simulink model "SistemaMasaResorteAmortiguadorDobleMasa"  (R2019a)
settings: Solver=VariableStepAuto  StartTime=0.0  StopTime=50  RelTol=1e-3
settings Model: Creator=User  LastModifiedBy=User

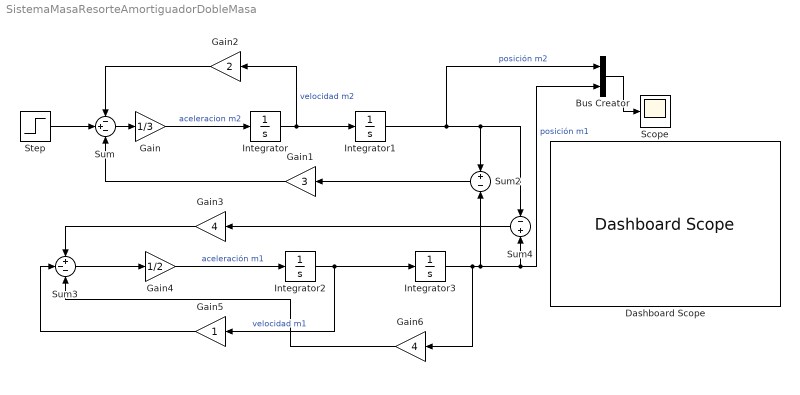
== system SistemaMasaResorteAmortiguadorDobleMasa ==
  Bus Creator : BusCreator  Inputs=2
  Dashboard Scope : DashboardScope
  Gain : Gain  Gain=1/3
  Gain1 : Gain  Gain=3
  Gain2 : Gain  Gain=2
  Gain3 : Gain  Gain=4
  Gain4 : Gain  Gain=1/2
  Gain5 : Gain
  Gain6 : Gain  Gain=4
  Integrator{,1..3} (4 alike) : Integrator
  Scope : Scope
  Step : Step  SampleTime=0
  Sum : Sum  Inputs=-+-
  Sum2 : Sum  Inputs=+-
  Sum3 : Sum  Inputs=+--
  Sum4 : Sum  Inputs=-+
  wires:
  Step/1 -> Sum/2
  Gain/1 -> Integrator/1  "aceleracion m2"
  Integrator/1 -> Integrator1/1, Gain2/1  "velocidad m2"
  Gain2/1 -> Sum/1
  Integrator1/1 -> Bus Creator/1, Sum4/1, Sum2/1  "posición m2"
  Gain1/1 -> Sum/3
  Gain3/1 -> Sum3/1
  Sum3/1 -> Gain4/1
  Sum2/1 -> Gain1/1
  Gain4/1 -> Integrator2/1  "aceleración m1"
  Integrator2/1 -> Integrator3/1, Gain5/1  "velocidad m1"
  Integrator3/1 -> Bus Creator/2, Sum4/2, Sum2/2, Gain6/1  "posición m1"
  Bus Creator/1 -> Scope/1
  Sum4/1 -> Gain3/1
  Sum/1 -> Gain/1
  Gain5/1 -> Sum3/2
  Gain6/1 -> Sum3/3
